simulink model "sampleModel1874"  (R2023a)
settings: Solver=VariableStepAuto  StartTime=0.0  StopTime=10.0  RelTol=1e-3
libraries: hdlsllib x10, simulink x1
settings Model: Creator=user1  LastModifiedBy=user1

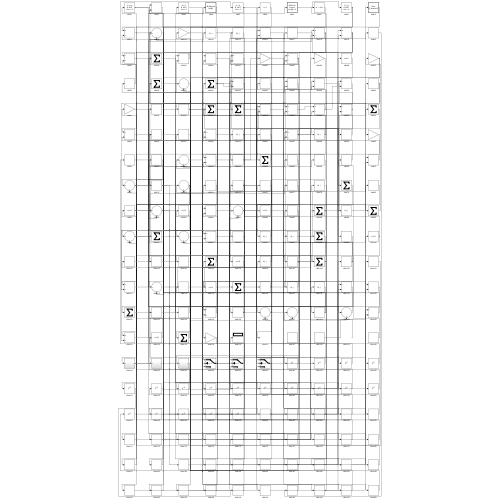
[thumbnail: Simulink's stored preview of the top-level diagram]
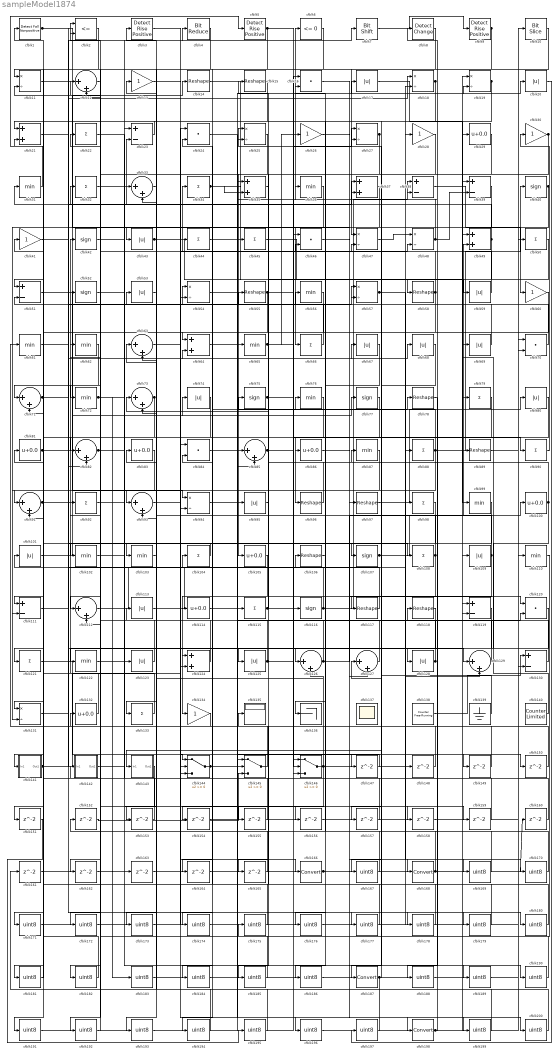
== system sampleModel1874 ==
  cfblk1 : hdlsllib/Logic and Bit Operations/Detect Fall Nonpositive  vinit=0  OutDataTypeStr=boolean
  cfblk10 : hdlsllib/Logic and Bit Operations/Bit Slice  lidx=7  ridx=0
  cfblk{29,81,83,86,100,105,114,132} (8 alike) : Bias  Bias=0.0  SaturateOnIntegerOverflow=off
  cfblk{17,20,43,53,59,67..69,74,80,95,101,109,113,123,125,128} (17 alike) : Abs  SaturateOnIntegerOverflow=off
  cfblk{31,36,56,61..62,65,72,76,87,99,102..103,110,122} (14 alike) : MinMax
  cfblk{22,32,34,44..45,50,66,79,88,90,92,98,104,108,115,121,133} (17 alike) : Sum  Inputs=+
  cfblk{14..15,55,58,78,89,96..97,106,117..118} (11 alike) : Reshape
  cfblk{40,42,52,75,77,107,116} (7 alike) : Signum
  cfblk{11,18..19,25,27,47..48,54,57,94,131} (11 alike) : Product  Inputs=*/  RndMeth=Zero  SaturateOnIntegerOverflow=on
  cfblk{23,38..39,51,111,119,130} (7 alike) : Sum  Inputs=+-
  cfblk{12,33,63,71,73,82,85,91,93,112,126..127,129} (13 alike) : Sum  Inputs=|++
  cfblk{16,24,46,70,84,120} (6 alike) : DotProduct  OutDataTypeStr=Inherit: Inherit via internal rule
  cfblk{21,35,37,49,64,124} (6 alike) : Sum
  cfblk{13,26,28,30,41,60,134} (7 alike) : Gain
  cfblk135 : Display
  cfblk136 : Terminator
  cfblk137 : Scope
      settings: Floating=on
  cfblk138 : hdlsllib/Sources/Counter Free-Running  NumBits=16  tsamp=-1
  cfblk139 : Ground
  cfblk140 : hdlsllib/Sources/Counter Limited  uplimit=7  tsamp=-1
  cfblk141 : Subsystem
      settings: LibrarySourceBlock=|
      | hdlsllib/Ports &
      | Subsystems/Subsystem
  cfblk142 : Subsystem
      settings: LibrarySourceBlock=|
      | hdlsllib/Ports &
      | Subsystems/Subsystem
  cfblk143 : Subsystem
      settings: LibrarySourceBlock=|
      | hdlsllib/Ports &
      | Subsystems/Subsystem
  cfblk144 : Switch  SaturateOnIntegerOverflow=off  InputSameDT=off
  cfblk145 : Switch  SaturateOnIntegerOverflow=off  InputSameDT=off
  cfblk146 : Switch  SaturateOnIntegerOverflow=off  InputSameDT=off
  cfblk{147..165} (19 alike) : Delay  SampleTime=1
  cfblk{166,168,187,198} (4 alike) : DataTypeConversion  SaturateOnIntegerOverflow=off  RndMeth=Floor
  cfblk{167,169..186,188..197,199..200} (31 alike) : DataTypeConversion  OutDataTypeStr=uint8  SaturateOnIntegerOverflow=off  RndMeth=Floor
  cfblk2 : RelationalOperator  Operator=<=  OutDataTypeStr=boolean  InputSameDT=off
  cfblk3 : hdlsllib/Logic and Bit Operations/Detect Rise Positive  vinit=0  OutDataTypeStr=boolean
  cfblk4 : hdlsllib/Logic and Bit Operations/Bit Reduce  mode=AND
  cfblk5 : hdlsllib/Logic and Bit Operations/Detect Rise Positive  vinit=0  OutDataTypeStr=boolean
  cfblk6 : hdlsllib/Logic and Bit Operations/Compare To Zero  relop=<=  OutDataTypeStr=boolean
  cfblk7 : hdlsllib/Logic and Bit Operations/Bit Shift  mode=Shift Left Logical  N=0
  cfblk8 : simulink/Logic and Bit Operations/Detect Change  vinit=0  OutDataTypeStr=boolean
      settings: LibrarySourceBlock=|
      | hdlsllib/Logic and Bit
      | Operations/Detect
      | Change
  cfblk9 : hdlsllib/Logic and Bit Operations/Detect Rise Positive  vinit=0  OutDataTypeStr=boolean
  wires:
  cfblk97/1 -> cfblk80/1
  cfblk2/1 -> cfblk11/1
  cfblk108/1 -> cfblk32/1, cfblk154/1
  cfblk116/1 -> cfblk38/1, cfblk75/1
  cfblk25/1 -> cfblk105/1
  cfblk9/1 -> cfblk71/1, cfblk51/1
  cfblk69/1 -> cfblk55/1
  cfblk104/1 -> cfblk103/1
  cfblk58/1 -> cfblk34/1, cfblk136/1, cfblk37/2
  cfblk95/1 -> cfblk104/1
  cfblk138/1 -> cfblk130/1
  cfblk96/1 -> cfblk73/1
  cfblk31/1 -> cfblk5/1
  cfblk105/1 -> cfblk134/1
  cfblk106/1 -> cfblk76/1
  cfblk127/1 -> cfblk73/2
  cfblk32/1 -> cfblk23/2
  cfblk54/1 -> cfblk20/1
  cfblk100/1 -> cfblk143/1(In1), cfblk15/1
  cfblk123/1 -> cfblk101/1
  cfblk40/1 -> cfblk131/2, cfblk181/1
  cfblk101/1 -> cfblk77/1
  cfblk72/1 -> cfblk7/1, cfblk163/1
  cfblk10/1 -> cfblk47/1
  cfblk7/1 -> cfblk9/1
  cfblk134/1 -> cfblk61/1
  cfblk118/1 -> cfblk187/1
  cfblk27/1 -> cfblk64/1, cfblk25/2
  cfblk91/1 -> cfblk14/1, cfblk57/1
  cfblk47/1 -> cfblk48/1
  cfblk23/1 -> cfblk21/1
  cfblk45/1 -> cfblk58/1
  cfblk112/1 -> cfblk85/1
  cfblk76/1 -> cfblk133/1
  cfblk129/1 -> cfblk11/2
  cfblk36/1 -> cfblk145/2
  cfblk63/1 -> cfblk198/1
  cfblk88/1 -> cfblk40/1, cfblk44/1, cfblk112/2
  cfblk132/1 -> cfblk71/2
  cfblk44/1 -> cfblk115/1
  cfblk39/1 -> cfblk66/1
  cfblk121/1 -> cfblk144/1
  cfblk107/1 -> cfblk49/2, cfblk170/1
  cfblk57/1 -> cfblk59/1, cfblk129/2
  cfblk77/1 -> cfblk96/1
  cfblk144/1 -> cfblk120/2, cfblk178/1
  cfblk82/1 -> cfblk126/1, cfblk183/1
  cfblk51/1 -> cfblk94/1
  cfblk133/1 -> cfblk42/1
  cfblk109/1 -> cfblk47/2, cfblk51/2, cfblk164/1
  cfblk124/1 -> cfblk52/1
  cfblk48/1 -> cfblk6/1, cfblk39/2
  cfblk139/1 -> cfblk87/1
  cfblk22/1 -> cfblk123/1
  cfblk81/1 -> cfblk67/1, cfblk107/1
  cfblk73/1 -> cfblk111/1, cfblk141/1(In1)
  cfblk140/1 -> cfblk69/1
  cfblk3/1 -> cfblk166/1
  cfblk120/1 -> cfblk122/1
  cfblk114/1 -> cfblk78/1
  cfblk89/1 -> cfblk10/1
  cfblk141/1(Out1) -> cfblk94/2, cfblk106/1
  cfblk11/1 -> cfblk97/1
  cfblk14/1 -> cfblk79/1
  cfblk90/1 -> cfblk30/1
  cfblk19/1 -> cfblk72/1, cfblk86/1, cfblk167/1
  cfblk8/1 -> cfblk82/1
  cfblk126/1 -> cfblk54/1, cfblk100/1
  cfblk113/1 -> cfblk88/1
  cfblk125/1 -> cfblk116/1, cfblk2/2
  cfblk122/1 -> cfblk64/2
  cfblk16/1 -> cfblk168/1
  cfblk6/1 -> cfblk124/1
  cfblk84/1 -> cfblk36/1
  cfblk1/1 -> cfblk45/1, cfblk124/2
  cfblk66/1 -> cfblk22/1
  cfblk80/1 -> cfblk121/1
  cfblk75/1 -> cfblk17/1, cfblk90/1, cfblk95/1, cfblk165/1
  cfblk21/1 -> cfblk128/1
  cfblk29/1 -> cfblk54/2
  cfblk37/1 -> cfblk112/1
  cfblk86/1 -> cfblk120/1
  cfblk79/1 -> cfblk144/3
  cfblk30/1 -> cfblk102/1, cfblk65/1
  cfblk18/1 -> cfblk43/1, cfblk114/1
  cfblk145/1 -> cfblk132/1
  cfblk70/1 -> cfblk27/1
  cfblk93/1 -> cfblk48/2
  cfblk59/1 -> cfblk12/1
  cfblk55/1 -> cfblk131/1, cfblk129/1
  cfblk49/1 -> cfblk117/1, cfblk31/1
  cfblk61/1 -> cfblk82/2
  cfblk131/1 -> cfblk4/1
  cfblk35/1 -> cfblk125/1
  cfblk5/1 -> cfblk108/1, cfblk153/1
  cfblk74/1 -> cfblk91/1
  cfblk85/1 -> cfblk149/1, cfblk150/1
  cfblk38/1 -> cfblk60/1
  cfblk34/1 -> cfblk146/2, cfblk35/2
  cfblk71/1 -> cfblk18/1, cfblk37/1
  cfblk43/1 -> cfblk99/1, cfblk127/2
  cfblk65/1 -> cfblk27/2, cfblk26/1
  cfblk128/1 -> cfblk56/1, cfblk93/2
  cfblk87/1 -> cfblk111/2
  cfblk102/1 -> cfblk74/1
  cfblk111/1 -> cfblk68/1
  cfblk103/1 -> cfblk53/1
  cfblk115/1 -> cfblk25/1, cfblk19/2
  cfblk146/1 -> cfblk113/1, cfblk18/2, cfblk184/1, cfblk186/1
  cfblk130/1 -> cfblk38/2
  cfblk117/1 -> cfblk2/1
  cfblk53/1 -> cfblk93/1
  cfblk17/1 -> cfblk89/1
  cfblk83/1 -> cfblk91/2
  cfblk64/1 -> cfblk147/1
  cfblk147/1 -> cfblk144/2
  cfblk148/1 -> cfblk84/2
  cfblk149/1 -> cfblk126/2
  cfblk150/1 -> cfblk46/2
  cfblk15/1 -> cfblk151/1
  cfblk152/1 -> cfblk145/3
  cfblk153/1 -> cfblk12/2
  cfblk154/1 -> cfblk49/1
  cfblk56/1 -> cfblk155/1
  cfblk155/1 -> cfblk23/1
  cfblk52/1 -> cfblk156/1
  cfblk156/1 -> cfblk70/2
  cfblk68/1 -> cfblk157/1
  cfblk157/1 -> cfblk1/1
  cfblk94/1 -> cfblk158/1
  cfblk158/1 -> cfblk39/1
  cfblk142/1(Out1) -> cfblk159/1
  cfblk159/1 -> cfblk145/1
  cfblk160/1 -> cfblk57/2
  cfblk161/1 -> cfblk146/3
  cfblk4/1 -> cfblk162/1
  cfblk162/1 -> cfblk146/1
  cfblk163/1 -> cfblk19/1
  cfblk165/1 -> cfblk35/1
  cfblk166/1 -> cfblk29/1, cfblk199/1
  cfblk167/1 -> cfblk3/1
  cfblk168/1 -> cfblk160/1, cfblk142/1(In1)
  cfblk26/1 -> cfblk169/1
  cfblk169/1 -> cfblk16/1
  cfblk170/1 -> cfblk16/2
  cfblk98/1 -> cfblk171/1
  cfblk171/1 -> cfblk84/1
  cfblk12/1 -> cfblk172/1
  cfblk172/1 -> cfblk98/1
  cfblk28/1 -> cfblk173/1
  cfblk173/1 -> cfblk148/1
  cfblk60/1 -> cfblk174/1
  cfblk174/1 -> cfblk28/1
  cfblk110/1 -> cfblk175/1
  cfblk175/1 -> cfblk152/1
  cfblk67/1 -> cfblk176/1
  cfblk176/1 -> cfblk110/1
  cfblk24/1 -> cfblk177/1
  cfblk177/1 -> cfblk135/1
  cfblk178/1 -> cfblk24/1
  cfblk42/1 -> cfblk179/1
  cfblk179/1 -> cfblk24/2
  cfblk41/1 -> cfblk180/1
  cfblk180/1 -> cfblk21/2
  cfblk181/1 -> cfblk41/1
  cfblk119/1 -> cfblk182/1
  cfblk182/1 -> cfblk81/1
  cfblk183/1 -> cfblk119/1
  cfblk184/1 -> cfblk119/2
  cfblk50/1 -> cfblk185/1
  cfblk185/1 -> cfblk83/1
  cfblk186/1 -> cfblk50/1
  cfblk187/1 -> cfblk161/1, cfblk127/1
  cfblk78/1 -> cfblk188/1
  cfblk188/1 -> cfblk118/1
  cfblk92/1 -> cfblk189/1
  cfblk189/1 -> cfblk70/1
  cfblk46/1 -> cfblk190/1
  cfblk190/1 -> cfblk92/1
  cfblk62/1 -> cfblk191/1
  cfblk191/1 -> cfblk85/2
  cfblk143/1(Out1) -> cfblk192/1
  cfblk192/1 -> cfblk62/1
  cfblk33/1 -> cfblk193/1
  cfblk193/1 -> cfblk46/1
  cfblk99/1 -> cfblk194/1
  cfblk194/1 -> cfblk33/1
  cfblk151/1 -> cfblk195/1
  cfblk195/1 -> cfblk33/2
  cfblk13/1 -> cfblk196/1
  cfblk196/1 -> cfblk130/2
  cfblk20/1 -> cfblk197/1
  cfblk197/1 -> cfblk13/1
  cfblk198/1 -> cfblk109/1, cfblk8/1
  cfblk199/1 -> cfblk63/1
  cfblk164/1 -> cfblk200/1
  cfblk200/1 -> cfblk63/2

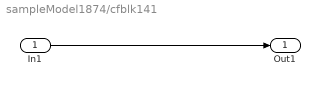
== system sampleModel1874/cfblk141 ==
  In1 : Inport
  Out1 : Outport
  wires:
  In1/1 -> Out1/1

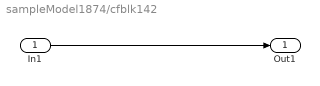
== system sampleModel1874/cfblk142 ==
  In1 : Inport
  Out1 : Outport
  wires:
  In1/1 -> Out1/1

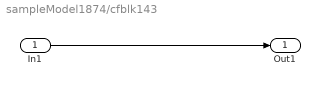
== system sampleModel1874/cfblk143 ==
  In1 : Inport
  Out1 : Outport
  wires:
  In1/1 -> Out1/1
